simulink model "Alone"  (Simulink 7.7)
settings: Solver=ode45  StartTime=0.0  StopTime=10.0  RelTol=1e-3
undefined symbols (not defined in the file or in its folder): gray
libraries: vipsnks x1, dspsrcs4 x1, vipconversions x1
settings Model: Creator=katsikas  LastModifiedBy=katsikas

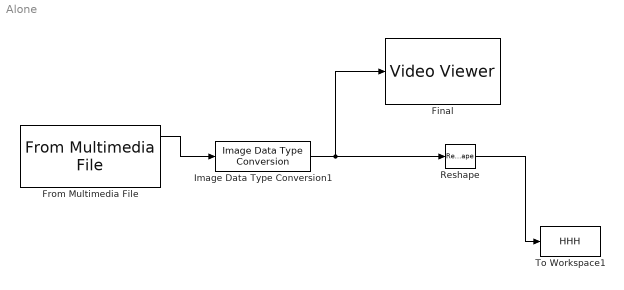
== system Alone ==
  Final : vipsnks/Video Viewer  inputType=Obsolete7b  imagePorts=One multidimensional signal  useColorMap=off  colormapValue=gray(256)  specRange=off  minInputVal=0  maxInputVal=255  FigPos=[765 683 237 300]  AxisZoom=on  trueSizedOnce=on  OpenAtMdlStart=on
  From Multimedia File : dspsrcs4/From Multimedia File  inputFilename=/home/katsikas/katsikas-repo/output.avi  loop=on  numPlays=inf  outputStreams=Video only  videoDataType=single  audioDataType=int16  inheritSampleTime=on  userDefinedSampleTime=1/30  noAudioOutput=off  isIntensityVideo=off  fourcc=YCbCr 4:2:2  colorVideoFormat=Separate color signals  outputEOF=off  dataOrg=Column-major  audioFrameSize=1024  computeAudioFrameSize=off
  Image Data Type Conversion1 : vipconversions/Image Data Type Conversion  outDT=single  isSigned=on  wordLen=16  numFracBits=0
  Reshape : Reshape  OutputDimensions=[19200,1]
  To Workspace1 : ToWorkspace  VariableName=HHH  SampleTime=-1  SaveFormat=Array
  wires:
  Image Data Type Conversion1/1 -> Final/1, Reshape/1
  Reshape/1 -> To Workspace1/1
  From Multimedia File/1 -> Image Data Type Conversion1/1
